simulink model "hmi_gfx_mgr02_if_model"  (Simulink 7.0)
settings: Solver=ode45  StartTime=0.0  StopTime=10.0  RelTol=1e-3
settings Model: Creator=emanoj1  LastModifiedBy=ashekhar

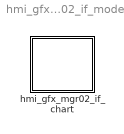
== system hmi_gfx_mgr02_if_model ==
  hmi_gfx_mgr02_if_chart : Stateflow chart

== stateflow chart hmi_gfx_mgr02_if_chart ==
  settings: executeAtInitialization=1
  state hmi_gfx_mgr02_if_shutdown(p_shutdown_type) [function]
    (junction 24) -> (junction 18) [order 2] : {
        |   GFX_MGR02_IF_DEACTIVATION_EV;
        | }
    (junction 24) -> (junction 25) [order 1] : [p_shutdown_type == GFX_MGR02_SHUTDOWN_EMERGENCY]
        | {
        | l_hm_emergency_shutdown_req = TRUE;
        | hmi_gfx_mgr02_emergency_shutdown();
        | }
    (default) -> (junction 24)
    (junction 34) -> (junction 18)
    (junction 25) -> (junction 34)
  state hmi_gfx_mgr02_if_KSTimedTask [function]
    (default) -> (junction 19)
    (junction 19) -> (junction 30) [order 2] : {
        |       GFX_MGR02_EXEC_EV;
        | }
    (junction 19) -> (junction 31) [order 1] : [l_hm_emergency_shutdown_req != FALSE]
        | {
        |     GFX_MGR02_IF_FORCED_DEACTIVATION_EV;
        | }
    (junction 35) -> (junction 30)
    (junction 31) -> (junction 35)
  state GFX_MGR02_IF_ST [parallel]
    entry:
    settings: executionOrder=2
    state GFX_MGR02_IF_SHUTDOWN_ST
      entry:
      hmi_gfx_mgr02_layout_shutdown();
    state GFX_MGR02_IF_TASK_ST
      en:
      l_hm_gt_tick_U8 = GFX_MGR02_IF_PRESENTATION_SCHED_COUNT;
      on GFX_MGR02_EXEC_EV:
      l_hm_gt_tick_U8 = (l_hm_gt_tick_U8+1);
      state GFX_MGR02_GT_WAIT_ST
        entry:
        l_hm_gt_tick_U8 = 0;
      state GFX_MGR02_REFRESH_WAIT_ST
      (default) -> (junction 20)
      (junction 20) -> GFX_MGR02_GT_WAIT_ST [order 1] : [in(GFX_MGR02_GT_BUSY_ST)]
      (junction 20) -> GFX_MGR02_REFRESH_WAIT_ST [order 2]
      GFX_MGR02_GT_WAIT_ST -> GFX_MGR02_REFRESH_WAIT_ST : GFX_MGR02_GT_DONE_EV
      GFX_MGR02_REFRESH_WAIT_ST -> (junction 40) : GFX_MGR02_EXEC_EV
          | [l_hm_gt_tick_U8 >= ...
          |      GFX_MGR02_IF_PRESENTATION_SCHED_COUNT]
      (junction 40) -> GFX_MGR02_GT_WAIT_ST [order 1] : [hmi_gfx_mgr02_if_presentation_task() != FALSE]
          | {
          |      send(GFX_MGR02_GT_EXECUTE_EV,GFX_MGR02_GT_ST);
          | }
      (junction 40) -> (junction 41) [order 2]
      (junction 41) -> GFX_MGR02_REFRESH_WAIT_ST : {
          |       l_hm_gt_tick_U8 = 0;
          | }
    state GFX_MGR02_IF_WAIT_ABNORMAL_SHUTDOWN_ST
    state GFX_MGR02_IF_WAIT_SHUTDOWN_ST
    (default) -> GFX_MGR02_IF_SHUTDOWN_ST
    (junction 23) -> GFX_MGR02_IF_SHUTDOWN_ST [order 2]
    GFX_MGR02_IF_SHUTDOWN_ST -> GFX_MGR02_IF_TASK_ST : GFX_MGR02_ACTIVATION_EV
        | {
        |    l_hm_emergency_shutdown_req = FALSE;
        |    hmi_gfx_mgr02_layout_initialize();
        |    hmi_gfx_mgr02_layout_startup();
        | }
    GFX_MGR02_IF_WAIT_ABNORMAL_SHUTDOWN_ST -> GFX_MGR02_IF_SHUTDOWN_ST : GFX_MGR02_GT_DONE_EV
    GFX_MGR02_IF_TASK_ST -> (junction 26) [order 1] : GFX_MGR02_IF_FORCED_DEACTIVATION_EV
    GFX_MGR02_IF_WAIT_SHUTDOWN_ST -> GFX_MGR02_IF_SHUTDOWN_ST [order 2] : GFX_MGR02_GT_DONE_EV
    (junction 26) -> GFX_MGR02_IF_WAIT_ABNORMAL_SHUTDOWN_ST [order 1] : [in(GFX_MGR02_GT_BUSY_ST)]
    (junction 26) -> GFX_MGR02_IF_SHUTDOWN_ST [order 2]
    GFX_MGR02_IF_TASK_ST -> (junction 23) [order 2] : GFX_MGR02_IF_DEACTIVATION_EV
    (junction 23) -> GFX_MGR02_IF_WAIT_SHUTDOWN_ST [order 1] : [in(GFX_MGR02_GT_BUSY_ST)]
    GFX_MGR02_IF_WAIT_SHUTDOWN_ST -> GFX_MGR02_IF_TASK_ST [order 3] : GFX_MGR02_ACTIVATION_EV
    GFX_MGR02_IF_WAIT_SHUTDOWN_ST -> GFX_MGR02_IF_WAIT_ABNORMAL_SHUTDOWN_ST [order 1] : GFX_MGR02_IF_FORCED_DEACTIVATION_EV
  state gfx_mgr02_start = hmi_gfx_mgr02_if_start [function]
    (default) -> (junction 21)
    (junction 21) -> (junction 38) [order 2]
    (junction 38) -> (junction 37) [order 1] : [in(GFX_MGR02_IF_WAIT_SHUTDOWN_ST) && (l_hm_emergency_shutdown_req == FALSE)]
        | {
        |   gfx_mgr02_start = TRUE;
        |   GFX_MGR02_ACTIVATION_EV;
        | }
    (junction 38) -> (junction 32) [order 2] : {
        | gfx_mgr02_start = FALSE;
        | }
    (junction 21) -> (junction 33) [order 1] : [in(GFX_MGR02_IF_SHUTDOWN_ST)]
        | {
        |   gfx_mgr02_start = TRUE;
        |   GFX_MGR02_ACTIVATION_EV;
        | }
    (junction 33) -> (junction 37)
    (junction 39) -> (junction 32)
    (junction 37) -> (junction 39)
  state Graphics_Task_Done [function]
    (default) -> (junction 22) : {
        |    GFX_MGR02_GT_DONE_EV;
        | }
  state ready_to_sleep = hmi_gfx_mgr02_if_is_ready_to_sleep [function]
    (junction 29) -> (junction 36)
    (junction 27) -> (junction 28) [order 2] : {
        | ready_to_sleep = FALSE;
        | }
    (default) -> (junction 27)
    (junction 27) -> (junction 29) [order 1] : [in(GFX_MGR02_IF_SHUTDOWN_ST)]
        | {
        | ready_to_sleep = TRUE;
        | }
    (junction 36) -> (junction 28)
  state GFX_MGR02_GT_ST [parallel]
    settings: executionOrder=1
    state GFX_MGR02_GT_IDLE_ST
    state GFX_MGR02_GT_BUSY_ST
    GFX_MGR02_GT_IDLE_ST -> GFX_MGR02_GT_BUSY_ST : GFX_MGR02_GT_EXECUTE_EV
    GFX_MGR02_GT_BUSY_ST -> GFX_MGR02_GT_IDLE_ST : GFX_MGR02_GT_DONE_EV
    (default) -> GFX_MGR02_GT_IDLE_ST
  data: p_shutdown_type function_input uint8; gfx_mgr02_start function_output uint8; ready_to_sleep function_output uint8; l_hm_gt_tick_U8 local uint8 =0; l_hm_emergency_shutdown_req local uint8 =0
  data l_hm_gt_tick_U8 settings: description=Indicates that presentation update request is active or not
  events: GFX_MGR02_ACTIVATION_EV local EITHER_EDGE_EVENT; GFX_MGR02_EXEC_EV local EITHER_EDGE_EVENT; GFX_MGR02_GT_DONE_EV local EITHER_EDGE_EVENT; GFX_MGR02_IF_DEACTIVATION_EV local EITHER_EDGE_EVENT; GFX_MGR02_IF_FORCED_DEACTIVATION_EV local EITHER_EDGE_EVENT; GFX_MGR02_GT_EXECUTE_EV local EITHER_EDGE_EVENT
